simulink model "Serial_Read"  (R2020a)
settings: Solver=FixedStepAuto  StartTime=0.0  StopTime=10.0  FixedStep=1e-3  RelTol=1e-3  EnableMultiTasking=on
undefined symbols (not defined in the file or in its folder): A0, A1, PTB2, PTB3
libraries: etargetslib x7, frdmk64flib x3
settings Model: ExtModeTrigDuration=5  Creator=iceca  LastModifiedBy=iceca
settings OptimizationCC: EnhancedBackFolding=on  PassReuseOutputArgsAs=Individual arguments  ZeroExternalMemoryAtStartup=off  ZeroInternalMemoryAtStartup=off  MaxStackSize=64  OptimizeBlockOrder=speed  DifferentSizesBufferReuse=on  OptimizationCustomize=off  EfficientTunableParamExpr=on
settings DebuggingCC: ParameterTunabilityLossMsg=error
settings HardwareCC: ProdBitPerPointer=32  ProdBitPerSizeT=32  ProdBitPerPtrDiffT=32  ProdLargestAtomicInteger=Long  ProdLargestAtomicFloat=Double  ProdWordSize=32  ProdHWDeviceType=ARM Compatible->ARM Cortex
settings SFSimCC: MATLABDynamicMemAlloc=off
settings RTWCC: SystemTargetFile=ert.tlc  HardwareBoard=NXP FRDM-K64F  TemplateMakefile=ert_default_tmf  Toolchain=GNU Tools for ARM Embedded Processors
settings CodeAppCC: ForceParamTrailComments=on  IgnoreCustomStorageClasses=off  OperatorAnnotations=on  SimulinkDataObjDesc=on  SFDataObjDesc=on  InsertBlockDesc=on

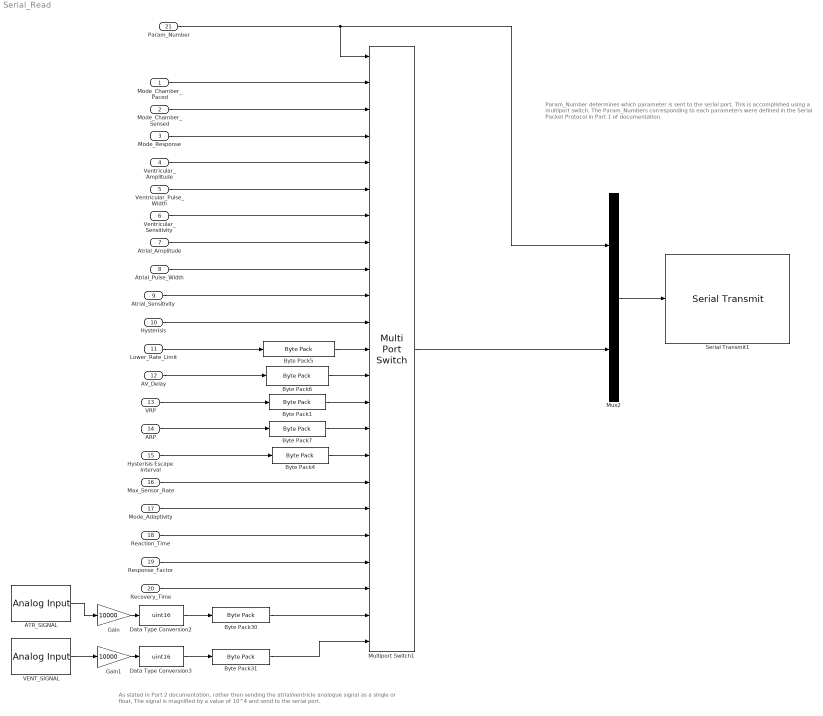
== system Serial_Read ==
  note: As stated in Part 2 documentation, rather then sending the atrial/ventricle analogue signal as a single or float,
      | The signal is magnified by a value of 10^4 and send to the serial port.
  note: Param_Number determines which parameter is sent to the serial port.
      | This is accomplished using a multiport switch.
      | The Param_Numbers corresponding to each parameters were defined in the
      | Serial Packet Protocol in Part 1 of documentation.
  Mode_Chamber_Paced : Inport  OutDataTypeStr=uint8
  Mode_Chamber_Sensed : Inport  Port=2  OutDataTypeStr=uint8
  Mode_Response : Inport  Port=3  OutDataTypeStr=uint8
  Ventricular_Amplitude : Inport  Port=4  OutDataTypeStr=uint8
  Ventricular_Pulse_Width : Inport  Port=5  OutDataTypeStr=uint8
  Ventricular_Sensitivity : Inport  Port=6  OutDataTypeStr=uint8
  Atrial_Amplitude : Inport  Port=7  OutDataTypeStr=uint8
  Atrial_Pulse_Width : Inport  Port=8  OutDataTypeStr=uint8
  Atrial_Sensitivity : Inport  Port=9  OutDataTypeStr=uint8
  Hysterisis : Inport  Port=10  OutDataTypeStr=uint8
  Lower_Rate_Limit : Inport  Port=11  OutDataTypeStr=uint16
  AV_Delay : Inport  Port=12  OutDataTypeStr=uint16
  VRP : Inport  Port=13  OutDataTypeStr=uint16
  ARP : Inport  Port=14  OutDataTypeStr=uint16
  Hysterisis Escape Interval : Inport  Port=15  OutDataTypeStr=uint16
  Max_Sensor_Rate : Inport  Port=16  OutDataTypeStr=uint8
  Mode_Adaptivity : Inport  Port=17  OutDataTypeStr=uint8
  Reaction_Time : Inport  Port=18  OutDataTypeStr=uint8
  Response_Factor : Inport  Port=19  OutDataTypeStr=uint8
  Recovery_Time : Inport  Port=20  OutDataTypeStr=uint8
  Param_Number : Inport  Port=21  OutDataTypeStr=uint8
  ATR_SIGNAL : frdmk64flib/Analog Input  Whichpin=PTB2 (A0)  SampleTime=-1
  Byte Pack{1,4..7,30..31} (7 alike) : etargetslib/Byte Pack  datatypes={'uint16'}  byteAlign=1
  Data Type Conversion2 : DataTypeConversion  OutDataTypeStr=uint16
  Data Type Conversion3 : DataTypeConversion  OutDataTypeStr=uint16
  Gain : Gain  Gain=10000
  Gain1 : Gain  Gain=10000
  Multiport Switch1 : MultiPortSwitch  Inputs=22
  Mux2 : Mux  Inputs=2
  Serial Transmit1 : frdmk64flib/Serial Transmit  SCIModule=0  Baudrate=uint32(9600)  Parity=None  StopBits=1  HardwareFlowControl=None  ByteOrder=LittleEndian  BlockingMode=on  OutputStatus=off
  VENT_SIGNAL : frdmk64flib/Analog Input  Whichpin=PTB3 (A1)  SampleTime=-1
  wires:
  Data Type Conversion2/1 -> Byte Pack30/1
  Data Type Conversion3/1 -> Byte Pack31/1
  Byte Pack31/1 -> Multiport Switch1/23
  VENT_SIGNAL/1 -> Gain1/1
  Byte Pack30/1 -> Multiport Switch1/22
  Gain1/1 -> Data Type Conversion3/1
  Mux2/1 -> Serial Transmit1/1
  Mode_Chamber_Paced/1 -> Multiport Switch1/2
  Recovery_Time/1 -> Multiport Switch1/21
  AV_Delay/1 -> Byte Pack6/1
  Hysterisis/1 -> Multiport Switch1/11
  Byte Pack4/1 -> Multiport Switch1/16
  Multiport Switch1/1 -> Mux2/2
  Max_Sensor_Rate/1 -> Multiport Switch1/17
  Atrial_Sensitivity/1 -> Multiport Switch1/10
  Byte Pack6/1 -> Multiport Switch1/13
  ATR_SIGNAL/1 -> Gain/1
  Mode_Chamber_Sensed/1 -> Multiport Switch1/3
  Param_Number/1 -> Mux2/1, Multiport Switch1/1
  VRP/1 -> Byte Pack1/1
  Byte Pack1/1 -> Multiport Switch1/14
  Mode_Response/1 -> Multiport Switch1/4
  Ventricular_Pulse_Width/1 -> Multiport Switch1/6
  Byte Pack7/1 -> Multiport Switch1/15
  Hysterisis Escape Interval/1 -> Byte Pack4/1
  Mode_Adaptivity/1 -> Multiport Switch1/18
  Reaction_Time/1 -> Multiport Switch1/19
  Byte Pack5/1 -> Multiport Switch1/12
  Atrial_Amplitude/1 -> Multiport Switch1/8
  Ventricular_Sensitivity/1 -> Multiport Switch1/7
  Ventricular_Amplitude/1 -> Multiport Switch1/5
  Atrial_Pulse_Width/1 -> Multiport Switch1/9
  Gain/1 -> Data Type Conversion2/1
  Lower_Rate_Limit/1 -> Byte Pack5/1
  ARP/1 -> Byte Pack7/1
  Response_Factor/1 -> Multiport Switch1/20
